simulink model "kr_billiards_demo2017"  (R2017a)
settings: Solver=VariableStepAuto  StartTime=0.0  StopTime=40  RelTol=1e-3  EnableMultiTasking=on
PreLoadFcn:
  | addpath('Bill_Tables_STEP')
  | addpath('Skins')
  | addpath('Utilities')
  | addpath('Kuka_KR10_R1100_STEP')
model workspace (MATLAB code in the model file):
  | den=1.613292710828678e+03;
  | st=0.004;
  | Damping=0.2;
  | 
  | % Length of brick solid
  | L = 20; % cm
  | % Width of brick solid
  | W = 2; % cm
  | % Height of brick solid
  | H = 2; % cm
  | % Density of brick solid
  | rho = 1000; % kg/m^3
undefined symbols (not defined in the file or in its folder): X, Y, Z
undefined symbols (not defined in the file): ball_col, ball_x, ball_y
libraries: sm_lib x83, nesl_utility x64, fl_lib x12, simulink x11
(part 4 of 4)

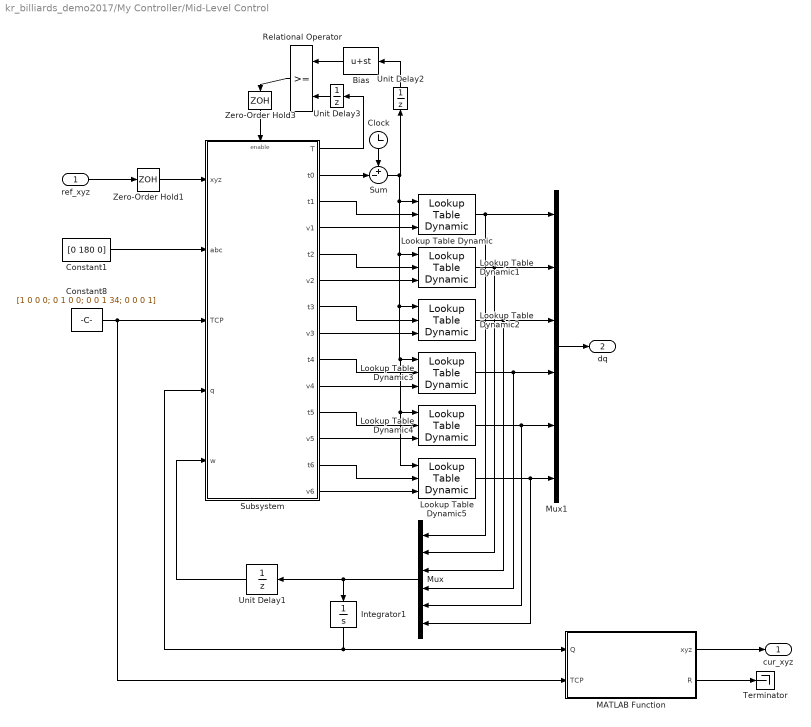
== system kr_billiards_demo2017/My Controller/Mid-Level Control ==
  ref_xyz : Inport
  Bias : Bias  Bias=st
  Clock : Clock
  Constant1 : Constant  Value=[0 180 0]
  Constant8 : Constant  Value=[1 0 0 0; 0 1 0 0; 0 0 1 34; 0 0 0 1]
  Integrator1 : Integrator
  Lookup Table Dynamic{,1..5} (6 alike) : simulink/Lookup Tables/Lookup Table Dynamic  LookUpMeth=Interpolation-Use End Values  OutDataType=fixdt('double')  OutScaling=[]  OutputDataTypeScalingMode=Specify via dialog  OutDataTypeStr=double  DoSatur=off
      settings: SourceProductName=Simulink
  MATLAB Function : MATLAB Function  TreatAsAtomicUnit=on
  Mux : Mux  Inputs=6
  Mux1 : Mux  Inputs=6
  Relational Operator : RelationalOperator  OutDataTypeStr=boolean  RndMeth=Simplest
  Subsystem : Subsystem
  Sum : Sum  Inputs=+-|
  Terminator : Terminator
  Unit Delay1 : UnitDelay  SampleTime=st
  Unit Delay2 : UnitDelay  SampleTime=st
  Unit Delay3 : UnitDelay  SampleTime=st
  Zero-Order Hold1 : ZeroOrderHold  SampleTime=st
  Zero-Order Hold3 : ZeroOrderHold  SampleTime=st
  cur_xyz : Outport
  dq : Outport  Port=2
  wires:
  Subsystem/9(t4) -> Lookup Table Dynamic3/2
  Subsystem/2(t0) -> Sum/2
  Subsystem/7(t3) -> Lookup Table Dynamic2/2
  Sum/1 -> Lookup Table Dynamic5/1, Lookup Table Dynamic4/1, Lookup Table Dynamic3/1, Lookup Table Dynamic2/1, Lookup Table Dynamic1/1, Lookup Table Dynamic/1, Unit Delay2/1
  Lookup Table Dynamic1/1 -> Mux1/2, Mux/2
  Clock/1 -> Sum/1
  Constant8/1 -> MATLAB Function/2(TCP), Subsystem/3(TCP)
  Subsystem/1(T) -> Unit Delay3/1
  Lookup Table Dynamic4/1 -> Mux1/5, Mux/5
  Subsystem/5(t2) -> Lookup Table Dynamic1/2
  Unit Delay3/1 -> Relational Operator/2
  Lookup Table Dynamic5/1 -> Mux1/6, Mux/6
  Unit Delay1/1 -> Subsystem/5(w)
  MATLAB Function/1(xyz) -> cur_xyz/1
  Mux1/1 -> dq/1
  Relational Operator/1 -> Zero-Order Hold3/1
  Lookup Table Dynamic2/1 -> Mux1/3, Mux/3
  Subsystem/8(v3) -> Lookup Table Dynamic2/3
  Subsystem/13(t6) -> Lookup Table Dynamic5/2
  Subsystem/12(v5) -> Lookup Table Dynamic4/3
  Subsystem/4(v1) -> Lookup Table Dynamic/3
  Mux/1 -> Integrator1/1, Unit Delay1/1
  Unit Delay2/1 -> Bias/1
  MATLAB Function/2(R) -> Terminator/1
  Subsystem/3(t1) -> Lookup Table Dynamic/2
  Subsystem/11(t5) -> Lookup Table Dynamic4/2
  Subsystem/14(v6) -> Lookup Table Dynamic5/3
  Subsystem/10(v4) -> Lookup Table Dynamic3/3
  Zero-Order Hold1/1 -> Subsystem/1(xyz)
  Lookup Table Dynamic/1 -> Mux1/1, Mux/1
  Subsystem/6(v2) -> Lookup Table Dynamic1/3
  Constant1/1 -> Subsystem/2(abc)
  ref_xyz/1 -> Zero-Order Hold1/1
  Zero-Order Hold3/1 -> Subsystem/Enable
  Lookup Table Dynamic3/1 -> Mux1/4, Mux/4
  Bias/1 -> Relational Operator/1
  Integrator1/1 -> Subsystem/4(q), MATLAB Function/1(Q)

== system kr_billiards_demo2017/My Controller/My Computer Vision ==
  cv_x : Inport
  cv_y : Inport  Port=2
  Detect Decrease2 : simulink/Logic and Bit Operations/Detect Decrease  vinit=0.0  OutDataTypeStr=boolean
  Detect Decrease3 : simulink/Logic and Bit Operations/Detect Decrease  vinit=0.0  OutDataTypeStr=boolean
  Step : Step  Time=20  Before=1  After=0  SampleTime=0
  Subsystem2 : Subsystem
      mask init:
      | numfoto = 5;
      | f = 500;
      | hx = 854;
      | hy = 480;
      | r = 34;         
      | 
      | load('cam_pos.mat','Q','TCP')
      | 
      | bg_rgb=[204 204 204];
      | tb_rgb=[2 157 41];
      | Bx=zeros(1,9);
      | By=Bx;
      | balls_found=0;
      | for n=1:numfoto
      |     imname=['image' num2str(n) '.bmp'];
      |     I=imread(imname);
      |     T=kuka_forward(Q(n,:),TCP);
      |     M=~(I(:,:,1)==bg_rgb(1) & I(:,:,2)==bg_rgb(2) & I(:,:,3)==bg_rgb(3)) & ~(I(:,:,1)==tb_rgb(1) & I(:,:,2)==tb_rgb(2) & I(:,:,3)==tb_rgb(3));
      |     s = regionprops(M,'Area','Centroid','MajorAxisLength','MinorAxisLength');
      |     for i=1:length(s)
      |         if s(i).Area>50 && abs(((s(i).MajorAxisLength-s(i).MinorAxisLength)/s(i).MajorAxisLength))<0.05 && abs(1-(1/16)*pi*(s(i).MajorAxisLength+s(i).MinorAxisLength)^2/s(i).Area)<0.05
      |             cam_r=sqrt((s(i).Area-sqrt(s(i).Area)*1.5)/pi);
      |             cam_z=f*r/cam_r;
      |             cam_x=cam_z*(s(i).Centroid(1)-hx/2)/f;
      |             cam_y=cam_z*(s(i).Centroid(2)-hy/2)/f;  
      |             ball_pos=T*[cam_x; cam_y; cam_z; 1];
      |             pos_x=ball_pos(1);
      |             pos_y=ball_pos(2);
      |             j=0;
      |             new_ball=true;
      |             while new_ball && j<balls_found 
      |                 j=j+1;
      |                 if sqrt((Bx(j)-pos_x)^2+(By(j)-pos_y)^2)<0.5*r
      |                     new_ball=false;
      |                     Bx(j)=(Bx(j)+pos_x)/2;
      |                     By(j)=(By(j)+pos_y)/2;
      |                 end
      |             end
      |             if new_ball
      |                 balls_found=balls_found+1;
      |                 Bx(balls_found)=pos_x;
      |                 By(balls_found)=pos_y;
      |             end
      |         end
      |     end
      | end
  Sum : Sum  Inputs=+
  Sum1 : Sum  Inputs=+
  Sum2 : Sum
  Switch : Switch  Criteria=u2 > Threshold
  Switch1 : Switch  Criteria=u2 > Threshold
  Zero-Order Hold2 : ZeroOrderHold  SampleTime=st
  Zero-Order Hold3 : ZeroOrderHold  SampleTime=st
  bx : Outport
  by : Outport  Port=2
  rst : Outport  Port=3
  wires:
  Switch/1 -> Zero-Order Hold2/1, by/1
  Subsystem2/1(Bx) -> Switch1/1
  Subsystem2/2(By) -> Switch/1
  Step/1 -> Switch/2, Switch1/2
  Switch1/1 -> bx/1, Zero-Order Hold3/1
  Detect Decrease2/1 -> Sum/1
  Sum/1 -> Sum2/1
  cv_x/1 -> Switch1/3
  Sum2/1 -> rst/1
  Zero-Order Hold3/1 -> Detect Decrease2/1
  cv_y/1 -> Switch/3
  Detect Decrease3/1 -> Sum1/1
  Sum1/1 -> Sum2/2
  Zero-Order Hold2/1 -> Detect Decrease3/1

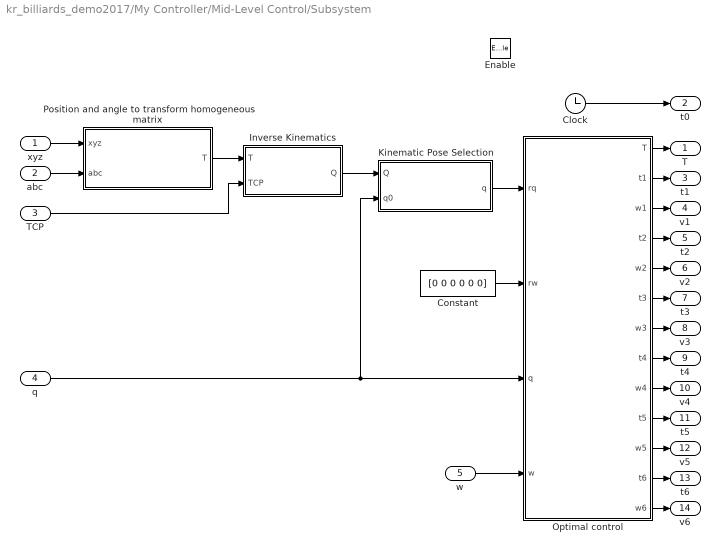
== system kr_billiards_demo2017/My Controller/Mid-Level Control/Subsystem ==
  xyz : Inport
  abc : Inport  Port=2
  TCP : Inport  Port=3
  q : Inport  Port=4
  w : Inport  Port=5
  Enable : EnablePort
  Clock : Clock
  Constant : Constant  Value=[0 0 0 0 0 0]
  Inverse Kinematics : MATLAB Function  TreatAsAtomicUnit=on
  Kinematic Pose Selection : MATLAB Function  TreatAsAtomicUnit=on
  Optimal control : MATLAB Function  TreatAsAtomicUnit=on
  Position and angle to transform homogeneous matrix : MATLAB Function  TreatAsAtomicUnit=on
  T : Outport
  t0 : Outport  Port=2
  t1 : Outport  Port=3
  v1 : Outport  Port=4
  t2 : Outport  Port=5
  v2 : Outport  Port=6
  t3 : Outport  Port=7
  v3 : Outport  Port=8
  t4 : Outport  Port=9
  v4 : Outport  Port=10
  t5 : Outport  Port=11
  v5 : Outport  Port=12
  t6 : Outport  Port=13
  v6 : Outport  Port=14
  wires:
  Kinematic Pose Selection/1(q) -> Optimal control/1(rq)
  Optimal control/6(t3) -> t3/1
  Optimal control/4(t2) -> t2/1
  Optimal control/9(w4) -> v4/1
  w/1 -> Optimal control/4(w)
  Optimal control/8(t4) -> t4/1
  Optimal control/11(w5) -> v5/1
  Optimal control/7(w3) -> v3/1
  Optimal control/2(t1) -> t1/1
  Optimal control/3(w1) -> v1/1
  Optimal control/12(t6) -> t6/1
  Optimal control/13(w6) -> v6/1
  Clock/1 -> t0/1
  Optimal control/1(T) -> T/1
  Optimal control/10(t5) -> t5/1
  Optimal control/5(w2) -> v2/1
  TCP/1 -> Inverse Kinematics/2(TCP)
  Position and angle to transform homogeneous matrix/1(T) -> Inverse Kinematics/1(T)
  xyz/1 -> Position and angle to transform homogeneous matrix/1(xyz)
  abc/1 -> Position and angle to transform homogeneous matrix/2(abc)
  Constant/1 -> Optimal control/2(rw)
  Inverse Kinematics/1(Q) -> Kinematic Pose Selection/1(Q)
  q/1 -> Kinematic Pose Selection/2(q0), Optimal control/3(q)

== system kr_billiards_demo2017/My Controller/My Computer Vision/Subsystem2 ==
  Constant1 : Constant  Value=By
  Constant2 : Constant  Value=Bx
  Bx : Outport
  By : Outport  Port=2
  wires:
  Constant2/1 -> Bx/1
  Constant1/1 -> By/1

== matlab function kr_billiards_demo2017/My Controller/Mid-Level Control/MATLAB Function ==
  data: Q input; xyz output; TCP input; R output
function [xyz, R]=kuka_forward(Q, TCP)
% Q - углы в осях, град
% TCP матрица однородного преобразования для инструмента (ориентация и положение в системе координат фланца)

% xyz - вектор положения работей точки манипулятора, заданной TCP
% R - матрица поворота инструмента


%% Параметры кинематической модели робота
% KUKA KR10 R1100
link1=400;
offset12=25;
link2=560;
offset23=35;
link34=515;
link56=80;

% % KUKA KR10 R900
% link2=455;
% link34=420;


Q=Q/180*pi;


%%

% матрица перехода от конечной точки робота до его фланца
F =[0 0 1 0; 0 1 0 0; -1 0 0 0; 0 0 0 1];

T1=[Rz(-Q(1)) [0 0 0 1]'];
T2=T1*[Ry(Q(2)) [offset12 0 link1 1]'];
T3=T2*[Ry(Q(3)) [link2 0 0 1]'];
T4=T3*[Rx(-Q(4)) [0 0 offset23 1]'];
T5=T4*[Ry(Q(5)) [link34 0 0 1]'];
T6=T5*[Rx(-Q(6)) [link56 0 0 1]'];
Tf=T6*F;
Tt=Tf*TCP;
xyz=Tt(1:3,4);
R=Tt(1:3,1:3);


    function R=Rx(q)
        R=[1,      0,       0;
            0, cos(q), -sin(q);
            0, sin(q),  cos(q);
            0,      0,      0];
    end


    function R=Ry(q)
        R=[cos(q)  0, sin(q);
            0     1,      0;
            -sin(q), 0, cos(q);
            0, 0,     0];
    end


    function R=Rz(q)
        R=[cos(q), -sin(q), 0;
            sin(q),  cos(q), 0;
            0,       0, 1;
            0,       0, 0];
    end
end

== matlab function kr_billiards_demo2017/My Controller/Mid-Level Control/Subsystem/Inverse Kinematics ==
  data: T input size=[4,4]; Q output size=[8,6]; TCP input size=[4,4]
function Q=inv_kin(T,TCP)
% npose - порядковый номер позы

% Принятые обозначения (система координат робота с началом в его основании):
% T - матрица перехода (матрица однородного преобразования) [4 x 4]
% R - матрица поворота [3 х 3], R = T(1:3, 1:3)
% P - вектор положения [3 x 1], P = T(1:3, 4)
% Индексы:
% 1..6 - звенья манипулятора (пример: R3 - матрица поворота третьего звена)
% f - фланец (пример: Pf - положение фланца)
%
% F - система координат фланца (начало в конечной точке манипулятора)
% TCP (Tool Center Point) - ориентация и положение инструмента в системе координат фланца (матрица однородного преобразования) [4 x 4]


%% Параметры кинематической модели робота
% KUKA KR10 R1100    
link1=400;
offset12=25;
link2=560;
offset23=35;
link34=515; 
link56=80; 

% % KUKA KR10 R900 
% link2=455;
% link34=420;

F =[0 0 1 0; 0 1 0 0; -1 0 0 0; 0 0 0 1];  % матрица перехода конечной точки манипулятора из глобальной системы координат в систему координат фланца 
%axlim=[-170 170; -190 45-40; -120 156; -185 185; -120 120; -350 350]*pi/180; % !!!! вторая ось доп. ограничена
% axspeed=[300 225 225 381 311 492];

%% 

% Обобщение звеньев 3 и 4 с учетом смещения offset23 (являются конструктивными константами для заданного типа манипулятора)
a=sqrt(offset23^2+link34^2);   % сторона A в теореме косинусов
b=link2;                       % сторона B в теореме косинусов
delta=atan2(offset23, link34); % угловая поправка 

Q=zeros(8,6);

% Переход от заданного положения TCP к соответствующему положению запястья  
Rf=T(1:3,1:3)*TCP(1:3,1:3)'; % система координат фланца в глобальной системе
P6=T(1:3,4)-Rf*TCP(1:3,4);   % положение конечной точки манипулятора в глобальной системе координат
R6=Rf*F(1:3,1:3)';           % ориентация конечной точки манипулятора в глобальной системе координат

% Координаты запястья (смещяемся от фланца до оси пятого шарнира по обратному направлению R6(:,1) (в системе координат робота в нулевой конфигурации он "вытянут" в направлении X)
x4=P6(1)-link56*R6(1,1);
y4=P6(2)-link56*R6(2,1);
z4=P6(3)-link56*R6(3,1);

L=sqrt(x4^2+y4^2); % длина проекции расстояния до заданной координаты запястья на плоскость xy в системе координат робота 

%% Ось 1
Q(1:4,1)=atan2(y4,x4);  % передом: угол "на цель"  % сингулярность, если y4=x4=0 
if Q(1,1)>0             % задом
    Q(5:8,1)=Q(1,1)-pi; 
else
    Q(5:8,1)=Q(1,1)+pi;
end 

%% Оси 2 и 3
% передом
[theta, alpha, gamma, ~] = angles_for_q123(L-offset12, z4-link1, a, b);
Q(1:2,2) = -theta-alpha;    % через верх (локототь вверх)
Q(1:2,3) = pi-gamma+delta;
Q(3:4,2) = -theta+alpha;    % через низ (локоть вниз)
Q(3:4,3) = -pi+gamma+delta;

% задом
[theta, alpha, gamma, ~] = angles_for_q123(L+offset12, z4-link1, a, b);
Q(5:6,2) = theta+alpha-pi;  % через верх (локототь вверх)
Q(5:6,3) = -pi+gamma+delta;
Q(7:8,2) = theta-alpha-pi;  % через низ (локоть вниз)
Q(7:8,3) = pi-gamma+delta;

%% Оси 4, 5, 6
for i=1:2:7
    [q4, q5, q6] = q456(Q(i,1), Q(i,2), Q(i,3), R6);
    Q(i:i+1,4)=q4;
    Q(i:i+1,5)=q5;
    Q(i:i+1,6)=q6;
end


% направление осей 1, 4 и 6 в роботе инвертировано
Q(:,1)=-Q(:,1);
Q(:,4)=-Q(:,4);
Q(:,6)=-Q(:,6);
Q=Q*180/pi;


function [q4, q5, q6] = q456(q1,q2,q3,R)
% Оси 4, 5, 6 для положительного и отрицательного угла в запястье
R = Ry(-q2-q3)*Rz(-q1)*R; % коррекция ориентации с учетом углов q1..q3
if R(1,1)<1
    q5 = [1; -1]*acos(R(1,1));
    q6 = atan2([1; -1]*R(1,2),[1; -1]*R(1,3));
    q4 = atan2([1; -1]*R(2,1),-[1; -1]*R(3,1));
else % вторая сингулярность 
    q5 = [0; 0];
    q4 = [0; 0];
    q6 = [1; 1]*atan2(R(3,2), R(3,3));   % atan2(R(3,2), R(3,3)); % сумма углов в осях 4 и 6
end


function [theta, alpha, gamma, ok] = angles_for_q123(L, z, a, b)
c = sqrt(L^2+z^2);            % сторона C в теореме косинусов
cos_alpha = (b^2+c^2-a^2)/(2*b*c);
cos_gamma = (a^2+b^2-c^2)/(2*a*b);
ok=true;
theta = atan2(z,L);             % наклон основания треугольника
if abs(cos_alpha)<=1
    alpha = acos(cos_alpha);    % угол альфа (в основании робота), берем действительную часть числа на случай, если cos>1
else
    alpha = (1-sign(cos_alpha))*pi/2;
    ok=false;
end
if abs(cos_gamma)<=1
    gamma = acos(cos_gamma);    % угол гамма (в локтевом шарнире)
else
    gamma = (1-sign(cos_gamma))*pi/2;
    ok=false;
end
    


function R=Ry(q)
R=[cos(q)  0, sin(q);
     0     1,      0;
  -sin(q), 0, cos(q)];


function R=Rz(q)
R=[cos(q), -sin(q), 0;
   sin(q),  cos(q), 0;
        0,       0, 1];

== matlab function kr_billiards_demo2017/My Controller/Mid-Level Control/Subsystem/Kinematic Pose Selection ==
  data: Q input size=[8,6]; q output size=[1,6]; q0 input size=[1,6]
function q = p_select(Q,q0)
%axlim=[-170 170; -190 45; -120 156; -185 185; -120 120; -350 350];   

n=1;
e_min=inf;
for i=1:8
    e=sum((Q(i,:) - q0).^2);
    if e<e_min
        e_min=e;
        n=i;
    end
end

q=Q(n,:);

== matlab function kr_billiards_demo2017/Billiards/MATLAB Function1 ==
  data: x0 input; y0 input; z0 input; x input; Fx output; y input; Fy output; U output
function [Fx, Fy, U] = fcn(x0, y0, z0, x, y)

R=0.034;  % радиус шара
%k=5000;
k=10000; % коэффициент упругости шар-шар
kb=10000; % коэффициент упругости борт-шар
kp=100; % коэффициент притяжения в центр лузы

RL=[0.1 0.1 0.065 0.1 0.1 0.065].^2;  % радиус луз в квадрате (из-за углубления угловые лузы "больше")


x_min=0.333;
x_max=1.116;
y_min=-0.8065;
y_max=0.8065;



s=0.051; % смещение лузы от борта 

% центры луз
Lx=[x_min-s x_max+s x_max+s x_max+s x_min-s x_min-s];
Ly=[y_max+s y_max+s 0 y_min-s y_min-s 0];


n=length(x);
Fx=zeros(n,1);
Fy=zeros(n,1);
z=0.103;  % 0.103 - уровень шаров по координате z 


U=zeros(n,1);  % 1 если шар в лузе

% попадания в лузы
for i=1:n
    for j=1:6
        dx=Lx(j)-x(i);
        dy=Ly(j)-y(i);
        if dx^2+dy^2<RL(j)
            U(i)=1;
            Fx(i)=dx*kp;
            Fy(i)=dy*kp;
        end
    end
    if U(i)==0 % если шар не в лузе, то проверяем удары об борта (упругий удар)
        Fx(i)=Fx(i)+kb*(x_min-x(i))*((x_min-x(i))>0)-kb*(x(i)-x_max)*((x(i)-x_max)>0);
        Fy(i)=Fy(i)+kb*(y_min-y(i))*((y_min-y(i))>0)-kb*(y(i)-y_max)*((y(i)-y_max)>0);       
    end
end


% биток по шарам
for i=1:n
    if U(i)==0
        dx=x0-x(i);
        dy=y0-y(i);
        r=sqrt(dx^2+dy^2+(z-z0)^2);
        d=r-2*R;
        if d<0
            Fx(i)=Fx(i)+k*d*dx/r;
            Fy(i)=Fy(i)+k*d*dy/r;
        end
    end
end



% соударения
for i=1:n-1
    if U(i)==0
        for j=i+1:n
            if U(j)==0
                dx=x(i)-x(j);
                dy=y(i)-y(j);
                r=sqrt(dx^2+dy^2);
                d=r-2*R;
                if d<0
                    fx=k*d*dx/r;
                    fy=k*d*dy/r;
                    Fx(i)=Fx(i)-fx;
                    Fx(j)=Fx(j)+fx;
                    Fy(i)=Fy(i)-fy;
                    Fy(j)=Fy(j)+fy;
                end
            end
        end
    end
end

== matlab function kr_billiards_demo2017/My Controller/Mid-Level Control/Subsystem/Optimal control ==
  settings: sampleTime=0.004
  data: T output; rq input size=6; t1 output size=[1 4]; rw input size=6; q input size=6; w input size=6; w1 output size=[1 4]; t2 output size=[1 4]; w2 output size=[1 4]; t3 output size=[1 4]; w3 output size=[1 4]; t4 output size=[1 4]; w4 output size=[1 4]; t5 output size=[1 4]; w5 output size=[1 4]; t6 output size=[1 4]; w6 output size=[1 4]
function [T,t1,w1,t2,w2,t3,w3,t4,w4,t5,w5,t6,w6] = opt_control(rq,rw,q,w)
%% Ввод данных
% q, w - текущее состояние (угол и угловая скорость)
% rq, rw  - заданное состояние (угол и угловая скорость)

vel_max = [300 225 225 381 311 492];       % максимальные скорости по осям
acc_max = vel_max*2;                       % максимальные ускорения по осям
%%
e=zeros(size(q));
time=e;
control_mode=true(size(q)); % true, если расчетная модель трехфазная 
for i=1:length(q)
    e(i) = rq(i) - q(i); % ошибка по углу
    % проверяем применимость трехфазной расчетной модели с выходом в насыщение по скорости
    v_max = sign(e(i)+eps)*vel_max(i);
    a_max = sign(e(i)+eps)*acc_max(i);
    time_a = (v_max-w(i))/a_max;
    time_b = (v_max-rw(i))/a_max;
    ab_rot = time_a*(w(i)+v_max)/2 + time_b*(rw(i)+v_max)/2;
    if abs(ab_rot) < abs(e(i))
        time_c = (e(i) - ab_rot)/v_max;
    else % если выход на постоянную (макс.) скорость отсвутсвует, то использем двухфазную расчетную модель
        control_mode(i)=false;
        time_c = 0;
        time_a = inf; time_b = inf;
        tmp1 = w(i)^2 + rw(i)^2;
        tmp2 = 2 * acc_max(i) * e(i);
        % Рассматриваем все 4 решения задачи и среди существующих выбираем с меньшим временем
        for z=[1 -1]                  % z=1: газ-тормоз / z=-1: тормоз-газ
            if tmp1+z*tmp2 >= 0
                d = sqrt((tmp1+z*tmp2)/2);
                % Решения #1 и #3 в зависимостт от z
                ta = -z*w(i) - d;
                tb = -z*rw(i) - d;
                if ta>=0 && tb>=0 && ta+tb<time_a+time_b
                    time_a=ta; time_b=tb;
                else % Решения #2 и #4 (здесь время всегда больше, чем в #1 и #4, т.к. здесь + d>0)
                    ta = -z*w(i) + d;
                    tb = -z*rw(i) + d;
                    if ta>=0 && tb>=0 && ta+tb<time_a+time_b
                        time_a=ta; time_b=tb;
                    end
                end
            end
        end
        time_a=time_a/acc_max(i);
        time_b=time_b/acc_max(i);
    end
    time(i)=time_a+time_b+time_c;
end
T=max(time);
if T<0.1
    T=0.1;
end

XDAT=zeros(6,4);
YDAT=zeros(6,4);

V_MAX=zeros(6,1);
ACC_A=zeros(6,1);
ACC_B=zeros(6,1);

for i=1:6
    OK=true(6,1);   
    tmp=w(i)+rw(i);
    tmp1=T^2*acc_max(i)^2-w(i)^2+2*w(i)*rw(i)-rw(i)^2;
    tmp2=acc_max(i)*(2*T*tmp-4*e(i));
    
    d=tmp1+tmp2;
    if d>-1e7
        if d<0
            d=0;
        else
            d=sqrt(d);
        end
        V_MAX(1) = (tmp+T*acc_max(i)+d)/2; ACC_A(1) = acc_max(i); ACC_B(1)= -acc_max(i);
        V_MAX(2) = (tmp+T*acc_max(i)-d)/2; ACC_A(2) = acc_max(i); ACC_B(2)= -acc_max(i);
    else
        OK(1:2)=false;
    end
    
    d=tmp1-tmp2;
    if d>-1e7
        if d<0
            d=0;
        else
            d=sqrt(d);
        end
        V_MAX(3) = (tmp-T*acc_max(i)+d)/2; ACC_A(3) = -acc_max(i); ACC_B(3)= acc_max(i);
        V_MAX(4) = (tmp-T*acc_max(i)-d)/2; ACC_A(4) = -acc_max(i); ACC_B(4)= acc_max(i);
    else
        OK(3:4)=false;
    end
    
    tmp = (w(i)^2-rw(i)^2)/2;
    tmp1 = w(i)-rw(i);
    tmp2 = tmp1+T*acc_max(i);
    if tmp2~=0
        V_MAX(5) = (tmp+acc_max(i)*e(i))/tmp2; ACC_A(5) = acc_max(i); ACC_B(5)= acc_max(i);
    else
        OK(5)=false;
    end
    tmp2 = tmp1-T*acc_max(i);
    if tmp2~=0
        V_MAX(6) = (tmp-acc_max(i)*e(i))/tmp2; ACC_A(6) = -acc_max(i); ACC_B(6)= -acc_max(i);
    else
        OK(6)=false;
    end
    j=0; stop=false;
    while j<6 && ~stop
        j=j+1;
        if OK(j)
            ta=(V_MAX(j)-w(i))/ACC_A(j); tb=(rw(i)-V_MAX(j))/ACC_B(j);
            if V_MAX(j)~=0
                tc = (e(i) - ta*(w(i)+V_MAX(j))/2 - tb*(rw(i)+V_MAX(j))/2)/V_MAX(j);
            else
                tc = T - ta - tb;
            end
            if ta>-1e-7 && tb>-1e-7 && tc>-1e-7
                if ta<0, ta=0; end
                if tc<0, tc=0; end
                xdat=[0 ta ta+tc T];
                ydat=[w(i) V_MAX(j) V_MAX(j) rw(i)];
                while ~all(diff(xdat)>eps)
                    if xdat(3)-xdat(2)<eps
                        if xdat(2)-xdat(1)<eps
                            sw1=3; sw2=4;
                        else
                            sw1=2; sw2=1;
                        end
                    elseif xdat(2)-xdat(1)<eps
                        sw1=2; sw2=3;
                    else
                        sw1=3; sw2=2;
                    end
                    xdat(sw1)=(xdat(sw1)+xdat(sw2))/2;
                    ydat(sw1)=(ydat(sw1)+ydat(sw2))/2;
                end
                XDAT(i,:)=xdat;
                YDAT(i,:)=ydat;
                stop=true;
            end
        end
    end
end
t1=XDAT(1,:); w1=YDAT(1,:);
t2=XDAT(2,:); w2=YDAT(2,:);
t3=XDAT(3,:); w3=YDAT(3,:);
t4=XDAT(4,:); w4=YDAT(4,:);
t5=XDAT(5,:); w5=YDAT(5,:);
t6=XDAT(6,:); w6=YDAT(6,:);

== matlab function kr_billiards_demo2017/My Controller/Mid-Level Control/Subsystem/Position and angle to transform homogeneous matrix ==
  data: xyz input; T output; abc input
function T = posang2transmat(xyz,abc)

a=abc(1)*pi/180;
b=abc(2)*pi/180;
c=abc(3)*pi/180;


Rx=[ 1, 0, 0;
     0, cos(c), -sin(c);
     0, sin(c), cos(c)];

Ry=[cos(b)  0, sin(b);
     0     1,      0;
  -sin(b), 0, cos(b)];

Rz=[cos(a), -sin(a), 0;
   sin(a),  cos(a), 0;
        0,       0, 1];
    

T=[[Rz*Ry*Rx; [0 0 0]], [reshape(xyz,3,1); 1]];

== matlab function kr_billiards_demo2017/My Controller/High-Level Control ==
  data: Robot_xyz input size=3; XYZ output; Ball_x input size=9; Ball_y input size=9; rst input; u input; u output
function [XYZ, u]  = fcn(Robot_xyz,Ball_x,Ball_y, rst,u)
% x,y,z - положение робота
% Bx, By - положение шаров на поле (вектор столбец из 9-ти элементов)
% VBx, VBy - скорости шаров (вектор столбец из 9-ти элементов)

Bx=Ball_x;
By=Ball_y;

if rst
    u(:)=1;
end

x=Robot_xyz(1);
y=Robot_xyz(2);
z=Robot_xyz(3);

% Положения бортов в системе координат робота 
x_min=333;
x_max=1116;
y_min=-806.5;
y_max=806.5;

s=51; % смещение лузы от борта 

% центры луз
Lx=[x_min-s x_max+s x_max+s x_max+s x_min-s x_min-s];
Ly=[y_max+s y_max+s 0 y_min-s y_min-s 0];

R=34;  % радиус шаров


%% Выбор целевого шара
nb=0;                                % порядковый номер ближайшего шара, если шар не найдется, то останентся nb=0 
r_min=inf;                          % инициализация значения целевой функции 
for i=1:length(Bx)
    if u(i)~=0 && Bx(i)>x_min && Bx(i)<x_max && By(i)>y_min && By(i)<y_max && sqrt(Bx(i)^2+By(i)^2)<1050 % если шар не в лузе и в поле досягаемости
        r=sqrt((Bx(i)-x).^2+(By(i)-y).^2); % расстояние от шара до битка
        if r<2*R
            u(i)=0;             % забываем про этот шар
        else
            if r<r_min          % выбираем шар по критерию минимума суммы квадрата расстояния до него и его модуля скорости
                r_min=r;
                nb=i;                    % порядковый номер ближайшего шара
            end
        end
    end
end

%rb=sqrt(r_min); % расстояние до целевого шара
rb=r_min;
%%
% nb - номер целевого шара
% np - номер целевой лузы
% tx - целевая координата по x
% ty - целевая координата по y

zdown=103;    % биток на уровене стола
zup=303;      % биток поднят на 200 мм для свободного перемещения над полем 

sens=1;      % чувствительность
runup=100;   % начальное расстояние между центрами битка и шара (разбег для удара)

ZD = z < zdown + sens;
ZU = z > zup - sens;

% 1. Есть два целевых уровня z: zdown=0.246 и zup=0.246+0.2 
% и два состония:  ZD = z < .247 - опущен, ZU = z > 0.245+0.2 - поднят

% 2. Есть расстояние до цели rt
% и факт ее достижения RT = rt < 0.001

% 3. Есть расстояние до центра мячика rb
% которое может быть меньше порога RB = rb < runup, когда шар гонят в лузу

% Если ZD && (RT || RB) то движемся в центр лузы np
% Ecли ~ZU && ~(RT || RB) не изменяя x и y, переводим z на уровень zup
% Ecли ZU && ~RT то двигаемся в tx и ty
% Ecли ~ZD && RT то опускаемся на уровени ZD 

tx=500;
ty=0; np=1;
if nb>0
    % Примеряемся к каждой из луз и выбираем ту, у которой исходная координата ближе 
    rt=inf;
    
    for i=1:length(Lx)
        dx=Lx(i)-Bx(nb);
        dy=Ly(i)-By(nb);
        r=sqrt(dx^2+dy^2);
        txi=Bx(nb)-runup*dx/r;        % исходная координата по x 
        tyi=By(nb)-runup*dy/r;        % исхолная координата по y 
        r=sqrt((txi-x)^2+(tyi-y)^2);
        if r<rt
            rt=r;                     % минимальное расстояние до исходной
            tx=txi;                   % ближайшая исходная по x
            ty=tyi;                   % ближайшая исходная по y
            np=i;                     % порядковый номер лузы
        end
    end
    RT = rt<sens;                     % биток в исходной точке на расстоянии разбега для удара (можно начинать движение в направлении удара) 
    RB = rb<runup;                    % биток ближе, чем разбег для удара (уже выполняется движение в направлении удара) 
    
    if ZD && (RT || RB)               % ЕСЛИ биток опущен и (достиг исходной точки или уже движется в сторну шара) 
        dx=Lx(np)-Bx(nb);
        dy=Ly(np)-By(nb);
        r=sqrt(dx^2+dy^2);      
        pos = [Bx(nb)-R*dx/r By(nb)-R*dy/r zdown];
    elseif ~ZU && ~(RT || RB)         % ЕСЛИ если биток не поднят и не (достиг исходной точки или уже движется в сторну шара)
        pos = [x y zup];              % ТО поднимаем биток веритикально, не меняя координат х и y
    elseif ZU && ~RT                  % ЕСЛИ биток поднят но не достиг исходной координаты  
        pos = [tx ty zup];            % ТО движемя в исходную координаиту (tx, ty) на высоте zup
    elseif ~ZD && RT                  % ЕСЛИ биток не опущен и достиг исходной точки 
        pos = [tx ty zdown];          % ТО сохораняем координату исходной точки и вертикально опускаем биток для удара  
    else                              % ИНАЧЕ
        pos = [500 0 zup];            % движемся в условный центр стола с поднятым битком   
    end
else
    pos = [tx ty zup];
end    
    
XYZ=pos;
